simulink library "Tire_Models"  (R2024a)
settings: Solver=VariableStepAuto  StartTime=0.0  StopTime=10.0  RelTol=1e-3
undefined symbols (not defined in the file): Vehicle, X, Y, Z
libraries: Tire_MFMbody x2, $bdroot x2, sm_lib x2
Description:
  | Copyright 2020-2023 The MathWorks, Inc.
settings Model: Creator=smiller  LastModifiedBy=lnicolet
settings SolverCC: AlgebraicLoopSolver=TrustRegion
settings DataIOCC: ReturnWorkspaceOutputs=off
settings OptimizationCC: ReuseModelBlockBuffer=off
settings DebuggingCC: UnconnectedInputMsg=warning  UnconnectedOutputMsg=warning  UnconnectedLineMsg=warning  ArithmeticOperatorsInVariantConditions=warning
settings ModelReferenceCC: EnableRefExpFcnMdlSchedulingChecks=on
settings SFSimCC: CustomCodeUndefinedFunction=UseInterfaceOnly
settings RTWCC: GPUComputeCapability=3.5  DLArmComputeVersion=19.05

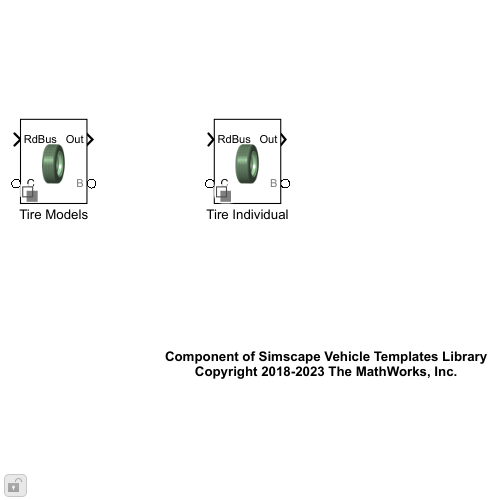
[thumbnail: Simulink's stored preview of the top-level diagram]
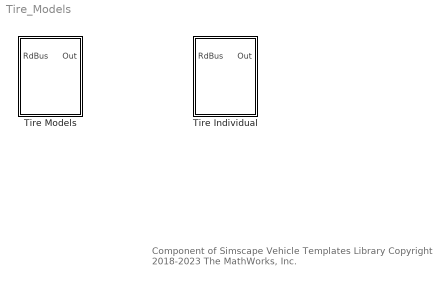
== system Tire_Models ==
  note: Component of Simscape Vehicle Templates Library
      | Copyright 2018-2023 The MathWorks, Inc.
  Tire Individual : Subsystem  Tag=PublishSubsystem  Variant=on  VariantControlMode=label  VariantControl=Variant1  LabelModeActiveChoice=MFMbody  mask(Tire){popup_leftRight=Right, tir_index=1, Tire=Vehicle.Chassis.TireA1, VariantLabel=Vehicle.Chassis.TireA1.class.Value, InitTriggerDropdown=1}
      mask prompts: popup_leftRight "Left/Right"; tir_index "Tire Index"; Tire "Tire Parameters"; VariantLabel "Variant Label"; InitTriggerDropdown "Initialization Trigger Dropdown"
      mask help: Configurable tire model.
      mask init:
      | curblk = gcb;
      | 
      | % Set variant for this block
      | set_param(curblk,'LabelModeActiveChoice',VariantLabel);
      | 
      | tir_variant = get_param(gcb,'ActiveVariant');
      | if (popup_leftRight == 1)
      |     if(strcmp(tir_variant,'MFEval'))
      |         set_param([gcb '/MFEval'],'tir_side','1 left');
      |         set_param([gcb '/MFEval'],'popup_leftRight','Left');
      |     elseif(strcmp(tir_variant,'CFL'))
      |         set_param([gcb '/CFL'],'popup_leftRight','Left');
      |     elseif(strcmp(tir_variant,'Testrig_Post'))
      |         set_param([gcb '/Testrig Post'],'popup_leftRight','Left');
      |     elseif(strcmp(tir_variant,'Delft'))
      |         set_param([gcb '/Delft'],'tire_side_mode','(1xxx) left');
      |         set_param([gcb '/Delft'],'popup_leftRight','Left');
      |     elseif(strcmp(tir_variant,'MFSwift'))
      |         set_param([gcb '/MFSwift'],'tire_side_mode','(x1xxx) left');
      |         set_param([gcb '/MFSwift'],'popup_leftRight','Left');
      |     elseif(strcmp(tir_variant,'MFMbody'))
      |         set_param([gcb '/MFMbody'],'tire_side','Left');
      |         set_param([gcb '/MFMbody'],'popup_leftRight','Left');        
      |     end
      | elseif (popup_leftRight == 2)
      |     if(strcmp(tir_variant,'MFEval'))
      |         set_param([gcb '/MFEval'],'tir_side','2 right');
      |         set_param([gcb '/MFEval'],'popup_leftRight','Right');
      |     elseif(strcmp(tir_variant,'CFL'))
      |         set_param([gcb '/CFL'],'popup_leftRight','Right');
      |     elseif(strcmp(tir_variant,'Testrig_Post'))
      |         set_param([gcb '/Testrig Post'],'popup_leftRight','Right');        
      |     elseif(strcmp(tir_variant,'Delft'))
      |         set_param([gcb '/Delft'],'tire_side_mode','(2xxx) right');
      |         set_param([gcb '/Delft'],'popup_leftRight','Right');
      |     elseif(strcmp(tir_variant,'MFSwift'))
      |         set_param([gcb '/MFSwift'],'tire_side_mode','(x2xxx) right');
      |         set_param([gcb '/MFSwift'],'popup_leftRight','Right');    
      |     elseif(strcmp(tir_variant,'MFMbody'))
      |         set_param([gcb '/MFMbody'],'tire_side','Right');
      |         set_param([gcb '/MFMbody'],'popup_leftRight','Right');
      |     end
      | end
      | 
      | % Trigger Mask Initialization for
      | % variant subsystems below this level
      | sm_car_lib_maskInitTrigger(curblk);
      settings: AttributesFormatString=%<ActiveVariant>
      mask TypeOptions popup_leftRight: Left | Right
      mask TypeOptions InitTriggerDropdown: 0 | 1
      mask Display:
      | switch lower(get_param(gcb,'LabelModeActiveChoice'))
      |     case 'mfeval', image('sm_car_vehicle_tire_mfeval_IMAGE.png');
      |     case 'delft', image('sm_car_vehicle_tire_delft_IMAGE.png');
      |     case 'mfswift', image('sm_car_vehicle_tire_delft_IMAGE.png');
      |     case 'mfmbody', image('sm_car_vehicle_tire_mfmbody_IMAGE.png');
      |     case 'cpi', image('sm_car_vehicle_tire_delftcpi_IMAGE.png');
      |     case 'cfl', image('sm_car_vehicle_tire_cfl_IMAGE.png');
      |     case 'testrig_post', image('sm_car_vehicle_tire_testrig_IMAGE.png');
      | end
  Tire Models : Subsystem  Tag=PublishSubsystem  Variant=on  VariantControlMode=label  VariantControl=Variant1  LabelModeActiveChoice=MFMbody  mask(Tire){popup_leftRight=Right, tir_index=1, Tire=Vehicle.Chassis.TireA1, VariantLabel=Vehicle.Chassis.TireA1.class.Value, InitTriggerDropdown=1}
      mask prompts: popup_leftRight "Left/Right"; tir_index "Tire Index"; Tire "Tire Parameters"; VariantLabel "Variant Label"; InitTriggerDropdown "Initialization Trigger Dropdown"
      mask help: Configurable tire model.
      mask init:
      | curblk = gcb;
      | 
      | % Set variant for this block 
      | set_param(curblk,'LabelModeActiveChoice',VariantLabel);
      | 
      | tir_variant = get_param(gcb,'ActiveVariant');
      | if (popup_leftRight == 1)
      |     rhs_tire = 1;
      |     if(strcmp(tir_variant,'MFEval'))
      |         set_param([gcb '/MFEval'],'tir_side','1 left');
      |         set_param([gcb '/MFEval'],'popup_leftRight','Left');
      |     elseif(strcmp(tir_variant,'Tire2x'))
      |         set_param([gcb '/Tire2x'],'popup_leftRight','Left');
      |     elseif(strcmp(tir_variant,'CFL'))
      |         set_param([gcb '/CFL'],'popup_leftRight','Left');
      |     elseif(strcmp(tir_variant,'Testrig_Post'))
      |         set_param([gcb '/Testrig Post'],'popup_leftRight','Left');
      |     elseif(strcmp(tir_variant,'Delft'))
      |         set_param([gcb '/Delft'],'tire_side_mode','(1xxx) left');
      |         set_param([gcb '/Delft'],'popup_leftRight','Left');
      |     elseif(strcmp(tir_variant,'MFSwift'))
      |         set_param([gcb '/MFSwift'],'tire_side_mode','(x1xxx) left');
      |         set_param([gcb '/MFSwift'],'popup_leftRight','Left');
      |     elseif(strcmp(tir_variant,'MFMbody'))
      |         set_param([gcb '/MFMbody'],'tire_side','Left');
      |         set_param([gcb '/MFMbody'],'popup_leftRight','Left');
      |     end
      | elseif (popup_leftRight == 2)
      |     rhs_tire = -1;
      |     if(strcmp(tir_variant,'MFEval'))
      |         set_param([gcb '/MFEval'],'tir_side','2 right');
      |         set_param([gcb '/MFEval'],'popup_leftRight','Right');
      |     elseif(strcmp(tir_variant,'Tire2x'))
      |         set_param([gcb '/Tire2x'],'popup_leftRight','Right');
      |     elseif(strcmp(tir_variant,'CFL'))
      |         set_param([gcb '/CFL'],'popup_leftRight','Right');
      |     elseif(strcmp(tir_variant,'Testrig_Post'))
      |         set_param([gcb '/Testrig Post'],'popup_leftRight','Right');
      |     elseif(strcmp(tir_variant,'Delft'))
      |         set_param([gcb '/Delft'],'tire_side_mode','(2xxx) right');
      |         set_param([gcb '/Delft'],'popup_leftRight','Right');
      |     elseif(strcmp(tir_variant,'MFSwift'))
      |         set_param([gcb '/MFSwift'],'tire_side_mode','(x2xxx) right');
      |         set_param([gcb '/MFSwift'],'popup_leftRight','Right');
      |     elseif(strcmp(tir_variant,'MFMbody'))
      |         set_param([gcb '/MFMbody'],'tire_side','Right');
      |         set_param([gcb '/MFMbody'],'popup_leftRight','Right');
      |         
      |     end
      | end
      | 
      | % Trigger Mask Initialization for 
      | % variant subsystems below this level
      | sm_car_lib_maskInitTrigger(curblk);
      settings: AttributesFormatString=%<ActiveVariant>
      mask TypeOptions popup_leftRight: Left | Right
      mask TypeOptions InitTriggerDropdown: 0 | 1
      mask Display:
      | switch lower(get_param(gcb,'LabelModeActiveChoice'))
      |     case 'mfeval', image('sm_car_vehicle_tire_mfeval_IMAGE.png');
      |     case 'delft', image('sm_car_vehicle_tire_delft_IMAGE.png');
      |     case 'mfmbody', image('sm_car_vehicle_tire_mfmbody_IMAGE.png');
      |     case 'mfswift', image('sm_car_vehicle_tire_delft_IMAGE.png');
      |     case 'cpi', image('sm_car_vehicle_tire_delftcpi_IMAGE.png');
      |     case 'cfl', image('sm_car_vehicle_tire_cfl_IMAGE.png');
      |     case 'testrig_post', image('sm_car_vehicle_tire_testrig_IMAGE.png');
      |     case 'tire2x',
      |         switch lower(get_param([gcb '/Tire2x/Tire Inner'],'LabelModeActiveChoice'))
      |             case 'mfeval', image('sm_car_vehicle_tire_mfeval2x_IMAGE.png');
      |             case 'delft', image('sm_car_vehicle_tire_delft2x_IMAGE.png');
      |             case 'mfswift', image('sm_car_vehicle_tire_delft2x_IMAGE.png');
      |             case 'mfmbody', image('sm_car_vehicle_tire_mfmbody2x_IMAGE.png');
      |             case 'cfl', image('sm_car_vehicle_tire_cfl2x_IMAGE.png');
      |             case 'testrig', image('sm_car_vehicle_tire_testrig2x_IMAGE.png');
      |         end
      | end

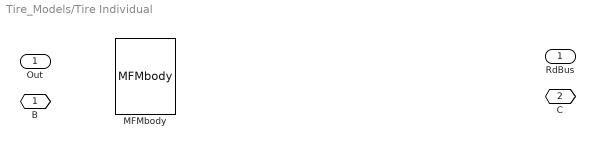
== system Tire_Models/Tire Individual ==
  RdBus : Inport
  MFMbody : Tire_MFMbody/MFMbody  VariantControl=MFMbody  tir_file=Tire.tirFile.Value  tire_side=Right  TireBody=Tire.TireBody  fcontactpatch=Tire.fContactPoint.Value  road_file=Tire.roadFile.Value  InitTriggerDropdown=1  popup_leftRight=Right  clr_tyre=Visual.Tire.clr  opc_tyre=Visual.Tire.opc  clr_rim=Visual.Rim.clr  opc_rim=Visual.Rim.opc
  " B" : PMIOPort  Side=Right
  " C" : PMIOPort  Port=2  Side=Left
  " Out" : Outport  VectorParamsAs1DForOutWhenUnconnected=off

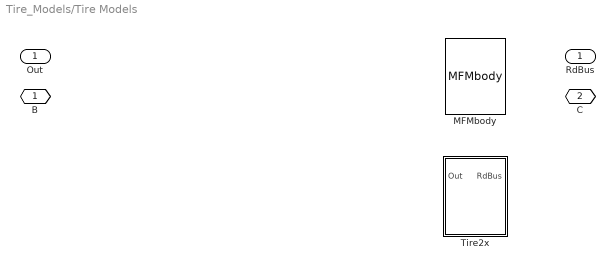
== system Tire_Models/Tire Models ==
  RdBus : Inport
  MFMbody : Tire_MFMbody/MFMbody  VariantControl=MFMbody  tir_file=Tire.tirFile.Value  tire_side=Right  TireBody=Tire.TireBody  fcontactpatch=Tire.fContactPoint.Value  road_file=Tire.roadFile.Value  InitTriggerDropdown=1  popup_leftRight=Right  clr_tyre=Visual.Tire.clr  opc_tyre=Visual.Tire.opc  clr_rim=Visual.Rim.clr  opc_rim=Visual.Rim.opc
  Tire2x : Subsystem  VariantControl=Tire2x  mask{popup_leftRight=Right, tir_index=tir_index, TireInner=Tire.TireInner, TireOuter=Tire.TireOuter, InitTriggerDropdown=1}
      mask prompts: popup_leftRight "Left/Right"; tir_index "Tire Index"; TireInner "Tire Inner (structure)"; TireOuter "Tire Outer (structure)"; InitTriggerDropdown "Initialization Trigger Dropdown"
      mask init:
      | curblk = gcb;
      | 
      | if(popup_leftRight == 1)
      |     set_param([curblk '/Tire Inner'],'popup_leftRight','Left');
      |     set_param([curblk '/Tire Outer'],'popup_leftRight','Left');
      | elseif(popup_leftRight == 2)
      |     set_param([curblk '/Tire Inner'],'popup_leftRight','Right');
      |     set_param([curblk '/Tire Outer'],'popup_leftRight','Right');
      | end
      | 
      | % Trigger Mask Initialization for 
      | % variant subsystems below this level
      | sm_car_lib_maskInitTrigger(curblk);
      mask TypeOptions popup_leftRight: Left | Right
      mask TypeOptions InitTriggerDropdown: 0 | 1
      mask DialogControl cont_tire_mfeval Prompt: Tire
  " B" : PMIOPort  Side=Right
  " C" : PMIOPort  Port=2  Side=Left
  " Out" : Outport  VectorParamsAs1DForOutWhenUnconnected=off

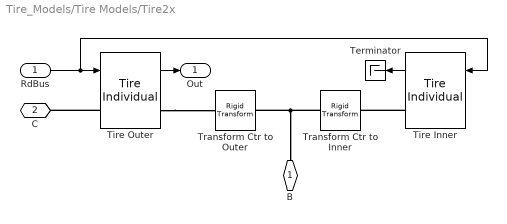
== system Tire_Models/Tire Models/Tire2x ==
  RdBus : Inport
  Terminator : Terminator
  Tire Inner : $bdroot/Tire Individual  Tag=PublishSubsystem  VariantControl=Variant1  LabelModeActiveChoice=MFMbody  popup_leftRight=Right  tir_index=tir_index+1  Tire=TireInner  VariantLabel=TireInner.class.Value  InitTriggerDropdown=1
      settings: AttributesFormatString=%<ActiveVariant>
  Tire Outer : $bdroot/Tire Individual  Tag=PublishSubsystem  VariantControl=Variant1  LabelModeActiveChoice=MFMbody  popup_leftRight=Right  tir_index=tir_index  Tire=TireOuter  VariantLabel=TireOuter.class.Value  InitTriggerDropdown=1
      settings: AttributesFormatString=%<ActiveVariant>
  Transform Ctr to Inner : sm_lib/Frames and Transforms/Rigid Transform  TranslationMethod=StandardAxis  TranslationStandardOffset=Tire.xOffset.Value/2*rhs_tire  TranslationStandardOffsetUnits=m  TranslationStandardAxis=-Z  TranslationCartesianOffset=[0 0 0]  TranslationCartesianOffsetUnits=m  TranslationROffset=0  TranslationROffsetUnits=m  TranslationZOffset=0  TranslationZOffsetUnits=m  TranslationThetaOffset=0  TranslationThetaOffsetUnits=deg  RotationMethod=None  RotationAngleUnits=deg  RotationStandardAxis=+Z  RotationAngle=0.0  RotationArbitraryAxis=[0 0 1]  FollAlignAxisA=+X  BaseAlignAxisA=+Y  FollAlignAxisB=+Y  BaseAlignAxisB=+Z  RotationSequenceAxes=FollowerAxes  RotationSequence=XYX  RotationSequenceAngles=[0 0 0]  RotationSequenceAnglesUnits=deg  RotationMatrix=[1 0 0; 0 1 0; 0 0 1]  Quaternion=[1 0 0 0]
  Transform Ctr to Outer : sm_lib/Frames and Transforms/Rigid Transform  TranslationMethod=StandardAxis  TranslationStandardOffset=Tire.xOffset.Value/2*rhs_tire  TranslationStandardOffsetUnits=m  TranslationStandardAxis=+Z  TranslationCartesianOffset=[0 0 0]  TranslationCartesianOffsetUnits=m  TranslationROffset=0  TranslationROffsetUnits=m  TranslationZOffset=0  TranslationZOffsetUnits=m  TranslationThetaOffset=0  TranslationThetaOffsetUnits=deg  RotationMethod=None  RotationAngleUnits=deg  RotationStandardAxis=+Z  RotationAngle=0.0  RotationArbitraryAxis=[0 0 1]  FollAlignAxisA=+X  BaseAlignAxisA=+Y  FollAlignAxisB=+Y  BaseAlignAxisB=+Z  RotationSequenceAxes=FollowerAxes  RotationSequence=XYX  RotationSequenceAngles=[0 0 0]  RotationSequenceAnglesUnits=deg  RotationMatrix=[1 0 0; 0 1 0; 0 0 1]  Quaternion=[1 0 0 0]
  B : PMIOPort  Side=Right
  C : PMIOPort  Port=2  Side=Left
  Out : Outport  VectorParamsAs1DForOutWhenUnconnected=off
  wires:
  RdBus/1 -> Tire Outer/1, Tire Inner/1
  Tire Outer/1 -> Out/1
  Tire Inner/1 -> Terminator/1
  connections:
  Transform Ctr to Inner/LConn1 -- B/RConn1 -- Transform Ctr to Outer/LConn1
  Tire Outer/LConn1 -- C/RConn1
  Tire Inner/RConn1 -- Transform Ctr to Inner/RConn1
  Tire Outer/RConn1 -- Transform Ctr to Outer/RConn1
